simulink library "NoiseModel_lib"  (Simulink 6.6)
undefined symbols (not defined in the file or in its folder): SensorNoise, Timestep
libraries: simulink x1
settings Model: Creator=cbuttril  LastModifiedBy=cbuttril

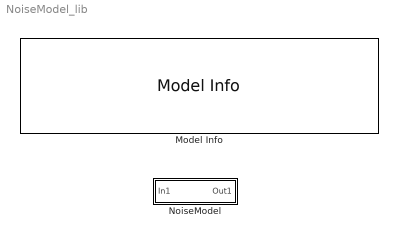
== system NoiseModel_lib ==
  Model Info : simulink/Model-Wide Utilities/Model Info  SystemSampleTime=-1  InitialBlockCM=None  BlockCM=None  Frame=on  DisplayStringWithTags=|  HorizontalTextAlignment=Center  LeftAlignmentValue=0.5  SourceBlockDiagram=NoiseModel_lib  TagMaxNumber=20
      | Developed using Matlab Release 2007a
      | 
      | SVN:%<ModelVersion>
      | Last modifed by %<LastModifiedBy> on %<LastModificationDate>
  NoiseModel : Subsystem  mask(Sensor Model){noise_on=SensorNoise.On, sigma=0, seed=878234, bias=0, scf=0}
      mask prompts: noise_on "on/off"; scf "scale factor:"
      mask help:
      | Add bias, scale factor, and white noise to a signal
      |
      | - 'on/off': 1 = noise on, 0 = noise off.
      | - 'sigma' : Standard deviation of white noise.
      | - 'seed'  : Random number seed. Generated numbers
      |   change between each simulation run, but the random number
      |   sequences do not change between Matlab sessions unless a
      |   new seed is specified.
      | - 'bias'  : Constant mean value offset of white noise.
      | - 'scale factor' : Scale factor applied to original signal.
      mask Display: disp('bias/scf/noise')

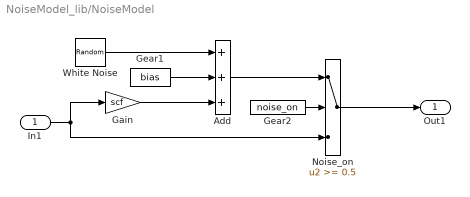
== system NoiseModel_lib/NoiseModel ==
  In1 : Inport
  Add : Sum  Inputs=+++  OutScaling=2^-10
  Gain : Gain  Gain=scf
  Gear1 : Constant  Value=bias
  Gear2 : Constant  Value=noise_on
  Noise_on : Switch  Threshold=0.5  SaturateOnIntegerOverflow=on  InputSameDT=on
  White Noise : RandomNumber  Variance=sigma*sigma  Seed=round(seed*rand(1))  SampleTime=Timestep
  Out1 : Outport
  wires:
  In1/1 -> Gain/1, Noise_on/3
  Gain/1 -> Add/3
  Gear1/1 -> Add/2
  Add/1 -> Noise_on/1
  White Noise/1 -> Add/1
  Gear2/1 -> Noise_on/2
  Noise_on/1 -> Out1/1
